simulink model "assignment7"  (R2019a)
settings: Solver=FixedStepDiscrete  StartTime=0.0  StopTime=10.0  RelTol=1e-3
libraries: simulink x1
settings Model: Creator=INDIA  LastModifiedBy=INDIA

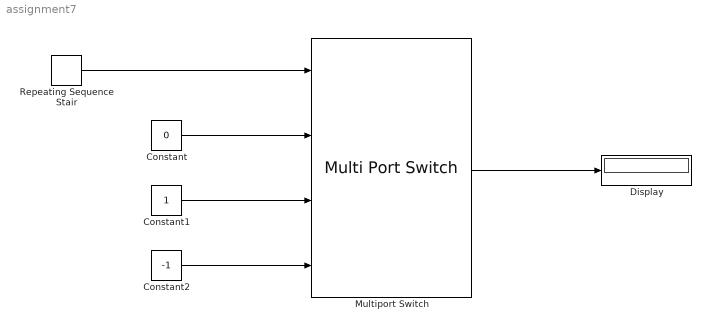
== system assignment7 ==
  Constant : Constant  Value=0
  Constant1 : Constant
  Constant2 : Constant  Value=-1
  Display : Display
  Multiport Switch : MultiPortSwitch  DataPortOrder=Specify indices  DataPortIndices={3,4,8}
  Repeating Sequence Stair : simulink/Sources/Repeating Sequence Stair  OutValues=[3 4 8 3 4 8 8 4 3 3 4].'  tsamp=-1  OutMin=[]  OutMax=[]  OutDataTypeStr=double  OutputDataTypeScalingMode=double  OutDataType=fixdt(0,8)  ConRadixGroup=Best Precision: Vector-wise  OutScaling=2^-12
  wires:
  Repeating Sequence Stair/1 -> Multiport Switch/1
  Constant1/1 -> Multiport Switch/3
  Constant/1 -> Multiport Switch/2
  Constant2/1 -> Multiport Switch/4
  Multiport Switch/1 -> Display/1
